simulink model "feedback_system"  (R2024a)
settings: Solver=ode45  StartTime=0.0  StopTime=300  MaxStep=1e-3  MinStep=1e-4  RelTol=1e-3
libraries: cstblocks x2
settings Model: Creator=larry  LastModifiedBy=larry
settings SolverCC: InitialStep=1e-4

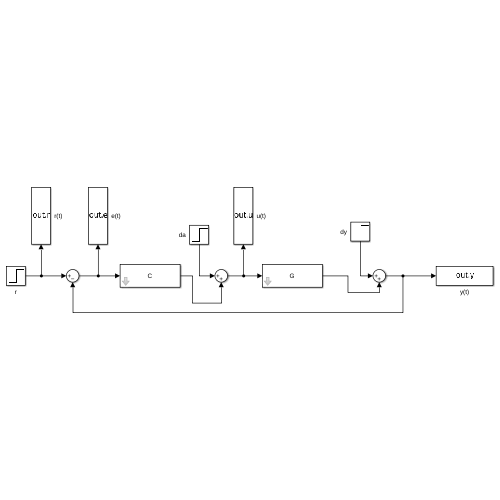
[thumbnail: Simulink's stored preview of the top-level diagram]
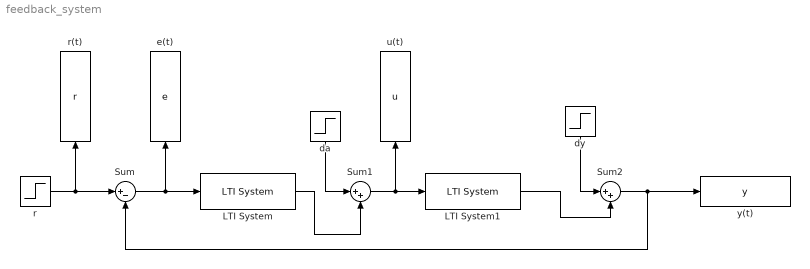
== system feedback_system ==
  LTI System : cstblocks/LTI System  sys=C  IC=[]  PadeOrder=0
  LTI System1 : cstblocks/LTI System  sys=G  IC=[]  PadeOrder=0
  Sum : Sum  Inputs=|+-
  Sum1 : Sum  Inputs=|++
  Sum2 : Sum  Inputs=|++
  da : Step  Time=0  After=0  SampleTime=0
  dy : Step  Time=0  After=0  SampleTime=0
  e(t) : ToWorkspace  VariableName=e  SaveFormat=Timeseries  SampleTime=-1
  r : Step  Time=0  SampleTime=0
  r(t) : ToWorkspace  VariableName=r  SaveFormat=Timeseries  SampleTime=-1
  u(t) : ToWorkspace  VariableName=u  SaveFormat=Timeseries  SampleTime=-1
  y(t) : ToWorkspace  VariableName=y  SaveFormat=Timeseries  SampleTime=-1
  wires:
  Sum/1 -> e(t)/1, LTI System/1
  LTI System1/1 -> Sum2/2
  r/1 -> Sum/1, r(t)/1
  LTI System/1 -> Sum1/2
  da/1 -> Sum1/1
  Sum1/1 -> u(t)/1, LTI System1/1
  dy/1 -> Sum2/1
  Sum2/1 -> y(t)/1, Sum/2
